simulink model "ParkAssist_Scenario001_cs"  (R2014b)
settings: Solver=ode5  SolverMode=SingleTasking  StartTime=0.0  StopTime=100  FixedStep=1/100  RelTol=1e-3
PreLoadFcn:
  | mbxruntime.callbacks.PreLoadFcn(bdroot);
  | check_NUTS_defined;
  | 
  | assignin('base',['model_closed_' bdroot],false);
  | addpath('../includes_AP');
PostLoadFcn:
  | mbxruntime.callbacks.PostLoadFcn(bdroot);
  | 
  | AP_PlotSpeed;
  | Sim_Stop();
InitFcn:
  | mbxruntime.callbacks.InitFcn(bdroot);
StartFcn:
  | mbxruntime.callbacks.StartFcn(bdroot);
StopFcn:
  | Sim_Stop();
  | 
  | mbxruntime.callbacks.StopFcn(bdroot);
model workspace: external: MAT-File .\ParkAssist_Scenario001_cs_hws.mat (data not in the file)
undefined symbols (not defined in the file or in its folder): mbxruntime, tabledata, warningInitialVelocity, x0
undefined symbols (not defined in the file): ParkAssist_Scenario001_cs_064fd3c184f1b23a, ParkAssist_Scenario001_cs_07cf59fafd9fba2a, ParkAssist_Scenario001_cs_0a672491f171a534, ParkAssist_Scenario001_cs_0b4ad32984af75f4, ParkAssist_Scenario001_cs_0d3d977035912083, ParkAssist_Scenario001_cs_10cfce74ee7f6e2a, ParkAssist_Scenario001_cs_10fa00b62d70eb48, ParkAssist_Scenario001_cs_1412412868c06c72, ParkAssist_Scenario001_cs_1415f498d2c97e5b, ParkAssist_Scenario001_cs_14cdb1b1e9831a61, ParkAssist_Scenario001_cs_17aa22f6296b2219, ParkAssist_Scenario001_cs_182e9fc64682f276, ParkAssist_Scenario001_cs_18d73450bb29fb11, ParkAssist_Scenario001_cs_1d2cd226ded8d576, ParkAssist_Scenario001_cs_1f257bc72917fbbc, ParkAssist_Scenario001_cs_1f636db8464e6ee8, ParkAssist_Scenario001_cs_20111ee9b4fc0884, ParkAssist_Scenario001_cs_20dc177d733a24ce, ParkAssist_Scenario001_cs_216ba491a5d003d6, ParkAssist_Scenario001_cs_23109d51cb4d704e, ParkAssist_Scenario001_cs_269c9790c06f4ab8, ParkAssist_Scenario001_cs_26fe2e7e8db3d6a5, ParkAssist_Scenario001_cs_29ddfbdf1c0505e3, ParkAssist_Scenario001_cs_2a5436d5f4ead3bb, ParkAssist_Scenario001_cs_2bb3c9b455f29773, ParkAssist_Scenario001_cs_2e8c42de3c2a47e4, ParkAssist_Scenario001_cs_31bf8e412bef9025, ParkAssist_Scenario001_cs_346fcd7bf176a778, ParkAssist_Scenario001_cs_3672d2bf8313cd6a, ParkAssist_Scenario001_cs_3741824a7a646254, ParkAssist_Scenario001_cs_39b3d14ce0df0209, ParkAssist_Scenario001_cs_3a61ee37372b31a8, ParkAssist_Scenario001_cs_3c92fe98e00232e8, ParkAssist_Scenario001_cs_3cb2af30b2d7797f, ParkAssist_Scenario001_cs_3cf6ddcf435d426b, ParkAssist_Scenario001_cs_3e68616cf9f62179, ParkAssist_Scenario001_cs_40255007183c2d89, ParkAssist_Scenario001_cs_453862d7bd596598, ParkAssist_Scenario001_cs_456f9ff24294bad4, ParkAssist_Scenario001_cs_45cf167d6b79cbb0, ParkAssist_Scenario001_cs_461748130c9c9c60, ParkAssist_Scenario001_cs_46b365d527226409, ParkAssist_Scenario001_cs_4cef5fe3be802cd9, ParkAssist_Scenario001_cs_4db296735c90de52, ParkAssist_Scenario001_cs_534e2bc3ff1a973e, ParkAssist_Scenario001_cs_55eebfeaa672d93d, ParkAssist_Scenario001_cs_585d6997c12221bd, ParkAssist_Scenario001_cs_5870adf5737dbe97, ParkAssist_Scenario001_cs_59a06d303da3d6df, ParkAssist_Scenario001_cs_59facc8727fc2440, ParkAssist_Scenario001_cs_5a3707b9202e3d67, ParkAssist_Scenario001_cs_5a9d74932f04a2aa, ParkAssist_Scenario001_cs_5b15da5d0cd6c04f, ParkAssist_Scenario001_cs_5cc17ff8d1eedb9f, ParkAssist_Scenario001_cs_5e786d0919c35899, ParkAssist_Scenario001_cs_60157af7bdca7094, ParkAssist_Scenario001_cs_6036a1ff9e25f439, ParkAssist_Scenario001_cs_6071b03654d6c39c, ParkAssist_Scenario001_cs_610f0d4aebe0cae1, ParkAssist_Scenario001_cs_622920b41ce6c5d3 ... (+103)
libraries: PreScanUsefulBlocks x57, PreScanSimulinkLibrary x56, simulink x55, simulink_extras x6
(part 9 of 15)

== system ParkAssist_Scenario001_cs/Audi_A8_1/AP_DEMO/Trigger_&_Display_Subsystem ==
  V [m/s] : Inport
  Gear : Inport  Port=2
  Throttle : Inport  Port=3
  Braking Pressure : Inport  Port=4
  Steering Angle : Inport  Port=5
  DISPLAY : M-S-Function  FunctionName=msfcn_AP_PlotSpeed  Parameters=DisplayFreq PathName
      mask Display:
      | port_label('input',1,'Velocity [km/h]');
      | port_label('input',2,'Gear');
      | port_label('input',3,'Brake Pressure [bar]');
      | port_label('input',4,'Throttle [%]');
      | port_label('input',5,'Steering Angle');
      | port_label('input',6,'Vehicle State');
  Error Check : Subsystem
  Rate Limiter : RateLimiter  RisingSlewLimit=500  FallingSlewLimit=-500  SampleTimeMode=inherited
  Trigger_system : Subsystem
  m/s 2 km/h : Gain  Gain=3.6
  Triggers : Outport
  Trigger2 : Outport  Port=2
  wires:
  Throttle/1 -> DISPLAY/4
  Braking Pressure/1 -> DISPLAY/3
  Steering Angle/1 -> Rate Limiter/1
  Gear/1 -> DISPLAY/2
  m/s 2 km/h/1 -> DISPLAY/1
  Trigger_system/2(Trigger2) -> Trigger2/1
  Trigger_system/1(Triggers) -> Triggers/1, DISPLAY/6
  V [m/s]/1 -> Trigger_system/1(V [m/s]), m/s 2 km/h/1
  Rate Limiter/1 -> DISPLAY/5

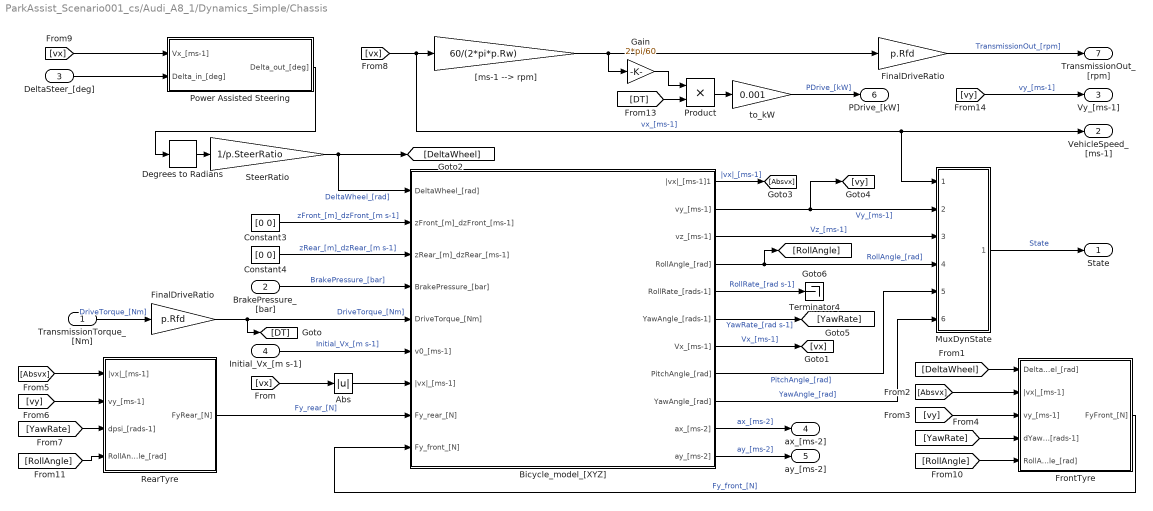
== system ParkAssist_Scenario001_cs/Audi_A8_1/Dynamics_Simple/Chassis ==
  TransmissionTorque_[Nm] : Inport
  BrakePressure_[bar] : Inport  Port=2
  DeltaSteer_[deg] : Inport  Port=3
  Initial_Vx_[m s-1] : Inport  Port=4
  Abs : Abs
  Bicycle_model_[XYZ] : Subsystem
      mask Display: image(imread('Bicycle_model.png'));
  Constant3 : Constant  Value=[0 0]
  Constant4 : Constant  Value=[0 0]
  Degrees to Radians : simulink_extras/Transformations/Degrees to Radians
  FinalDriveRatio : Gain  Gain=p.Rfd  SaturateOnIntegerOverflow=on  OutDataTypeStr=Inherit: Same as input  ParamDataTypeStr=Inherit: Same as input
  "FinalDriveRatio " : Gain  Gain=p.Rfd  SaturateOnIntegerOverflow=on  OutDataTypeStr=Inherit: Same as input  ParamDataTypeStr=Inherit: Same as input
  FrontTyre : Subsystem
      mask Display: image(imread('Tyre.png'));
  Gain : Gain  Gain=2*pi/60
  MuxDynState : Subsystem
  Power Assisted Steering : Subsystem
  Product : Product  RndMeth=Zero
  RearTyre : Subsystem
      mask Display: image(imread('Tyre.png'));
  SteerRatio : Gain  Gain=1/p.SteerRatio
  Terminator4 : Terminator
  "[ms-1 --> rpm]" : Gain  Gain=60/(2*pi*p.Rw)  SaturateOnIntegerOverflow=on  OutDataTypeStr=Inherit: Same as input  ParamDataTypeStr=Inherit: Same as input
  to_kW : Gain  Gain=0.001
  State : Outport
  VehicleSpeed_[ms-1] : Outport  Port=2
  Vy_[ms-1] : Outport  Port=3
  ax_[ms-2] : Outport  Port=4
  ay_[ms-2] : Outport  Port=5
  PDrive_[kW] : Outport  Port=6
  TransmissionOut_[rpm] : Outport  Port=7
  wires:
  [vy] -> Vy_[ms-1]/1  "vy_[ms-1]"
  to_kW/1 -> PDrive_[kW]/1  "PDrive_[kW]"
  Gain/1 -> Product/1
  Bicycle_model_[XYZ]/10(ax_[ms-2]) -> ax_[ms-2]/1  "ax_[ms-2]"
  Product/1 -> to_kW/1
  [DT] -> Product/2
  Bicycle_model_[XYZ]/11(ay_[ms-2]) -> ay_[ms-2]/1  "ay_[ms-2]"
  Abs/1 -> Bicycle_model_[XYZ]/7(|vx|_[ms-1])
  Degrees to Radians/1 -> SteerRatio/1
  [vx] -> Abs/1
  SteerRatio/1 -> [DeltaWheel], Bicycle_model_[XYZ]/1(DeltaWheel_[rad])  "DeltaWheel_[rad]"
  TransmissionTorque_[Nm]/1 -> "FinalDriveRatio "/1  "DriveTorque_[Nm]"
  RearTyre/1(FyRear_[N]) -> Bicycle_model_[XYZ]/8(Fy_rear_[N])  "Fy_rear_[N]"
  FrontTyre/1(FyFront_[N]) -> Bicycle_model_[XYZ]/9(Fy_front_[N])  "Fy_front_[N]"
  Bicycle_model_[XYZ]/1(|vx|_[ms-1]1) -> [Absvx]  "|vx|_[ms-1]"
  Bicycle_model_[XYZ]/2(vy_[ms-1]) -> [vy], MuxDynState/2(vy [ms-1])  "Vy_[ms-1]"
  Bicycle_model_[XYZ]/4(RollAngle_[rad]) -> MuxDynState/4(R [rad]), [RollAngle]  "RollAngle_[rad]"
  Bicycle_model_[XYZ]/6(YawAngle_[rads-1]) -> [YawRate]  "YawRate_[rad s-1]"
  Bicycle_model_[XYZ]/7(Vx_[ms-1]) -> [vx]  "Vx_[ms-1]"
  [DeltaWheel] -> FrontTyre/1(DeltaWheel_[rad])
  [Absvx] -> FrontTyre/2(|vx|_[ms-1])
  [vy] -> FrontTyre/3(vy_[ms-1])
  [YawRate] -> FrontTyre/4(dYawAngle_[rads-1])
  [Absvx] -> RearTyre/1(|vx|_[ms-1])
  [vy] -> RearTyre/2(vy_[ms-1])
  [YawRate] -> RearTyre/3(dpsi_[rads-1])
  Bicycle_model_[XYZ]/3(vz_[ms-1]) -> MuxDynState/3(vz [ms-1])  "Vz_[ms-1]"
  Bicycle_model_[XYZ]/8(PitchAngle_[rad]) -> MuxDynState/5(P [rad])  "PitchAngle_[rad]"
  Bicycle_model_[XYZ]/9(YawAngle_[rad]) -> MuxDynState/6(Y [rad])  "YawAngle_[rad]"
  "[ms-1 --> rpm]"/1 -> Gain/1, FinalDriveRatio/1
  FinalDriveRatio/1 -> TransmissionOut_[rpm]/1  "TransmissionOut_[rpm]"
  [vx] -> "[ms-1 --> rpm]"/1, VehicleSpeed_[ms-1]/1, MuxDynState/1(vx [ms-1])  "vx_[ms-1]"
  [vx] -> Power Assisted Steering/1(Vx_[ms-1])
  DeltaSteer_[deg]/1 -> Power Assisted Steering/2(Delta_in_[deg])
  Power Assisted Steering/1(Delta_out_[deg]) -> Degrees to Radians/1
  [RollAngle] -> FrontTyre/5(RollAngle_[rad])
  [RollAngle] -> RearTyre/4(RollAngle_[rad])
  Constant3/1 -> Bicycle_model_[XYZ]/2(zFront_[m]_dzFront_[ms-1])  "zFront_[m]_dzFront_[m s-1]"
  Constant4/1 -> Bicycle_model_[XYZ]/3(zRear_[m]_dzRear_[ms-1])  "zRear_[m]_dzRear_[m s-1]"
  BrakePressure_[bar]/1 -> Bicycle_model_[XYZ]/4(BrakePressure_[bar])  "BrakePressure_[bar]"
  "FinalDriveRatio "/1 -> Bicycle_model_[XYZ]/5(DriveTorque_[Nm]), [DT]  "DriveTorque_[Nm]"
  Initial_Vx_[m s-1]/1 -> Bicycle_model_[XYZ]/6(v0_[ms-1])  "Initial_Vx_[m s-1]"
  Bicycle_model_[XYZ]/5(RollRate_[rads-1]) -> Terminator4/1  "RollRate_[rad s-1]"
  MuxDynState/1(State) -> State/1  "State"

== system ParkAssist_Scenario001_cs/Audi_A8_1/Dynamics_Simple/Engine ==
  ImpellerTorque_[Nm] : Inport
  Throttle_[%] : Inport  Port=2
  Configurable Subsystem : Subsystem  BlockChoice=Discrete Rate Limiter  mask{ComputationMode=ComputationMode}
      mask prompts: ComputationMode "Compuation mode:"
      mask init:
      | SetComputationMode(gcb,ComputationMode);
      settings: AttributesFormatString=%<BlockChoice>  OpenFcn=BringToFront(gcb);  MemberBlocks=Discrete Rate Limiter,Rate Limiter
      settings: TemplateBlock=|
      | PreScanSimulinkLibrary/Configurable Subsystems/TransferFunction
      | Engine/Configurable
      | Subsystem
  Configurable Subsystem1 : Subsystem  BlockChoice=Discrete-Time Integrator  mask{ComputationMode=ComputationMode}
      mask prompts: ComputationMode "Computation mode:"
      mask init:
      | SetComputationMode(gcb,ComputationMode);
      settings: AttributesFormatString=%<BlockChoice>  OpenFcn=BringToFront(gcb);  MemberBlocks=Discrete-Time Integrator,Integrator
      settings: TemplateBlock=|
      | PreScanSimulinkLibrary/Configurable Subsystems/integral with initial condition and limts
      | for engine/Configurable
      | Subsystem
  EngineTorque : Lookup2D  RowIndex=p.thvec  ColumnIndex=p.nevec  Table=p.emap  InputSameDT=on
  Gain : Gain  Gain=2*pi/60
  Product : Product  RndMeth=Zero
  Sum : Sum  Inputs=-+  SaturateOnIntegerOverflow=on  InputSameDT=on  OutDataTypeStr=Inherit: Same as first input
  engine + impeller inertia : Gain  Gain=1/p.Iei  SaturateOnIntegerOverflow=on  OutDataTypeStr=Inherit: Same as input  ParamDataTypeStr=Inherit: Same as input
  rad|sec2rpm : Gain  Gain=60/2/pi  SaturateOnIntegerOverflow=on  OutDataTypeStr=Inherit: Same as input  ParamDataTypeStr=Inherit: Same as input
  to_kW : Gain  Gain=0.001
  nEngine_[rpm] : Outport  InitialOutput=0
  PEngine_[kW] : Outport  Port=2  InitialOutput=0
  wires:
  rad|sec2rpm/1 -> nEngine_[rpm]/1, EngineTorque/2, Gain/1  "rpm"
  engine + impeller inertia/1 -> Configurable Subsystem1/1(In1)  "rads-2"
  EngineTorque/1 -> Sum/2, Product/2
  Sum/1 -> engine + impeller inertia/1
  Configurable Subsystem1/1(Out1) -> rad|sec2rpm/1  "rads-1"
  Throttle_[%]/1 -> Configurable Subsystem/1(In1)
  ImpellerTorque_[Nm]/1 -> Sum/1
  Configurable Subsystem/1(Out1) -> EngineTorque/1
  Product/1 -> to_kW/1
  Gain/1 -> Product/1
  to_kW/1 -> PEngine_[kW]/1

== system ParkAssist_Scenario001_cs/Audi_A8_1/Dynamics_Simple/Gear: Auto Manual ==
  note: 0; Auto = on // Manual =off
      | 1; Auto = off // Manual =on
  Auto_Manual : Inport
  Manual_Gear : Inport  Port=2
  Auto_Gear : Inport  Port=3
  If : If  IfExpression=u1 == 0
  If Action Subsystem : Subsystem  TreatAsAtomicUnit=on
  If Action Subsystem1 : Subsystem  TreatAsAtomicUnit=on
  Merge : Merge
  Gear : Outport
  wires:
  If Action Subsystem/1(Out1) -> Merge/1
  Auto_Gear/1 -> If Action Subsystem/1(In1)
  If/1 -> If Action Subsystem/Action
  Merge/1 -> Gear/1
  If Action Subsystem1/1(Out1) -> Merge/2
  Manual_Gear/1 -> If Action Subsystem1/1(In1)
  If/2 -> If Action Subsystem1/Action
  Auto_Manual/1 -> If/1

== system ParkAssist_Scenario001_cs/Audi_A8_1/Dynamics_Simple/ShiftLogic ==
  Throttle_[%] : Inport
  GearNr_[-] : Inport  Port=2
  Auto_GearShift : Inport  Port=3
  VehSpeed_[ms-1] : Inport  Port=4
  Add2 : Sum
  Data Type Conversion1 : DataTypeConversion  OutDataTypeStr=double
  Detect Increase1 : simulink/Logic and Bit Operations/Detect Increase  vinit=0.0  InputProcessing=Inherited  OutDataTypeStr=uint8
  Detect Increase : Subsystem
  Gear limitation : Saturate  UpperLimit=p.maxGear  LowerLimit=1
  Gear limitation while shifting : Saturate  UpperLimit=p.maxGear  LowerLimit=1
  GearNeutral : Constant  Value=0
  GearReverse : Constant  Value=-1
  "IC, gear = 1" : Memory  X0=1  InheritSampleTime=on
  If Action Neutral : Subsystem  TreatAsAtomicUnit=on
  If Action Normal : Subsystem  TreatAsAtomicUnit=on
  If Action Reverse : Subsystem  TreatAsAtomicUnit=on
  Memory : Memory  InheritSampleTime=on
  Merge : Merge  Inputs=3
  Relational Operator : RelationalOperator  OutDataTypeStr=boolean
  Relational Operator1 : RelationalOperator  Operator=<=  OutDataTypeStr=boolean
  Shift_Down time : Delay  DelayLength=p.ShiftDown_fac  InputProcessing=Inherited
  Shift_Up time : Delay  DelayLength=p.ShiftUp_fac  InputProcessing=Inherited
  Sum : Sum  Inputs=+-
  interp_down : Lookup2D  RowIndex=p.downth  ColumnIndex=[1:p.maxGear]  Table=p.downtab  LookUpMeth=Interpolation-Use End Values  InputSameDT=on
  interp_up : Lookup2D  RowIndex=p.upth  ColumnIndex=[1:p.maxGear]  Table=p.uptab  LookUpMeth=Interpolation-Use End Values  InputSameDT=on
  reverse/neutral/normal gear : If  IfExpression=u1 == 0  ElseIfExpressions=u1 < 0
  to_ms-1 : Gain  Gain=1/3.6
  "to_ms-1 " : Gain  Gain=1/3.6
  GearNr : Outport
  wires:
  Auto_GearShift/1 -> reverse/neutral/normal gear/1
  "IC, gear = 1"/1 -> If Action Normal/1(In1)
  Merge/1 -> GearNr/1
  If Action Reverse/1(Out1) -> Merge/2
  If Action Neutral/1(Out1) -> Merge/1
  If Action Normal/1(Out1) -> Merge/3
  reverse/neutral/normal gear/3 -> If Action Normal/Action
  reverse/neutral/normal gear/1 -> If Action Neutral/Action
  reverse/neutral/normal gear/2 -> If Action Reverse/Action
  GearReverse/1 -> If Action Reverse/1(In1)
  GearNeutral/1 -> If Action Neutral/1(In1)
  Shift_Down time/1 -> Sum/2
  Shift_Up time/1 -> Sum/1
  Detect Increase/1(Out1) -> Shift_Up time/1
  Data Type Conversion1/1 -> Shift_Down time/1
  Detect Increase1/1 -> Data Type Conversion1/1
  Sum/1 -> Add2/1
  Memory/1 -> Add2/2  "GearNr_[-]"
  Add2/1 -> Gear limitation while shifting/1
  Gear limitation while shifting/1 -> "IC, gear = 1"/1, Memory/1  "GearNr_[-]"
  Throttle_[%]/1 -> interp_down/1, interp_up/1
  Relational Operator/1 -> Detect Increase/2(In2)
  Relational Operator1/1 -> Detect Increase1/1
  interp_down/1 -> "to_ms-1 "/1
  VehSpeed_[ms-1]/1 -> Relational Operator/1, Relational Operator1/1
  interp_up/1 -> to_ms-1/1
  Gear limitation/1 -> interp_down/2, interp_up/2, Detect Increase/1(GearNr_[-])
  GearNr_[-]/1 -> Gear limitation/1
  to_ms-1/1 -> Relational Operator/2
  "to_ms-1 "/1 -> Relational Operator1/2

== system ParkAssist_Scenario001_cs/Audi_A8_1/Dynamics_Simple/Transmission ==
  nEngine_[rpm] : Inport
  GearNr_[-] : Inport  Port=2
  n_TransmissionOut_[rpm] : Inport  Port=3
  Torque_Converter : Subsystem
      mask Display: image(imread('TorqueConverter.png'));
  Transmission_Ratio : Subsystem
  Viscous coupling : Lookup  InputValues=[-5:0.1:5]*p.m/4  Table=p.m/4*tanh([-5:0.1:5])
  ImpellerTorque_[Nm] : Outport  InitialOutput=0
  TransmissionTorque_[Nm] : Outport  Port=2  InitialOutput=0
  wires:
  Torque_Converter/2(TurbineTorque_[Nm]) -> Viscous coupling/1  "Converter_Torque_[Nm]"
  Transmission_Ratio/2(nTransmissionIn_[rpm]) -> Torque_Converter/2(nTransmission_[rpm])
  nEngine_[rpm]/1 -> Torque_Converter/1(nEngine_[rpm])
  GearNr_[-]/1 -> Transmission_Ratio/2(GearNr_[-]), Torque_Converter/3(Gear nr)
  n_TransmissionOut_[rpm]/1 -> Transmission_Ratio/3(nTransmissionOut_[rpm])
  Torque_Converter/1(ImpellerTorque_[Nm]) -> ImpellerTorque_[Nm]/1
  Transmission_Ratio/1(tTransmissionOut_[Nm]) -> TransmissionTorque_[Nm]/1
  Viscous coupling/1 -> Transmission_Ratio/1(tTransmissionIn_[Nm])

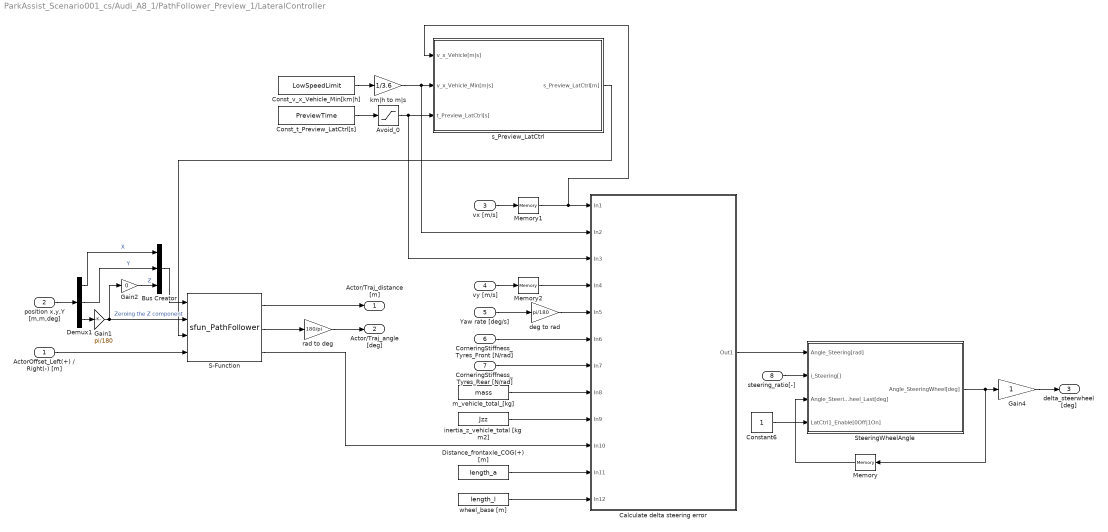
== system ParkAssist_Scenario001_cs/Audi_A8_1/PathFollower_Preview_1/LateralController ==
  ActorOffset_Left(+) / Right(-) [m] : Inport
  position x,y,Y [m,m,deg] : Inport  Port=2
  vx [m/s] : Inport  Port=3
  vy [m/s] : Inport  Port=4
  Yaw rate [deg/s] : Inport  Port=5
  CorneringStiffness_Tyres_Front [N/rad] : Inport  Port=6
  CorneringStiffness_Tyres_Rear [N/rad] : Inport  Port=7
  steering_ratio[-] : Inport  Port=8
  Avoid_0 : Saturate  UpperLimit=1000  LowerLimit=0.1
  Bus Creator : BusCreator  Inputs='X','Y','Z'  OutDataTypeStr=Bus: PRESCAN_XYZ_DATA
  Calculate delta steering error : Subsystem
      mask Display:
      | port_label('input', 1, 'v_x_vehicle [m/s]')
      | port_label('input', 2, 'v_x_vehicle_Min [m/s]')
      | port_label('input', 3, 't_Preview_LatCtrl [s]')
      | port_label('input', 4, 'v_y_vehicle [m/s]')
      | port_label('input', 5, 'yawrate_vehicle [rad/sec]')
      | port_label('input', 6, 'CorneringStiffness_Tyres_Front [N/rad]')
      | port_label('input', 7, 'CorneringStiffness_Tyres_Rear [N/rad]')
      | port_label('input', 8, 'm_vehicle_total [kg]')
      | port_label('input', 9, 'inertia_z_vehicle_total [kg m2]')
      | port_label('input', 10, 'e_Lat [m]')
      | port_label('input', 11, 'Distance_frontaxle_COG(+) [m]')
      | port_label('input', 12, 'wheel_base [m]')
      | port_label('output', 1, 'delta_steeringwheel [rad]')
  Const_t_Preview_LatCtrl[s] : Constant  Value=PreviewTime  SampleTime=CSSampleTime
  Const_v_x_Vehicle_Min[km|h] : Constant  Value=LowSpeedLimit  SampleTime=CSSampleTime
  Constant6 : Constant  SampleTime=CSSampleTime
  Demux1 : Demux  Outputs=3
  Distance_frontaxle_COG(+) [m] : Constant  Value=length_a  SampleTime=CSSampleTime
  Gain1 : Gain  Gain=pi/180
  Gain2 : Gain  Gain=0
  Gain4 : Gain
  Memory : Memory  InheritSampleTime=on
  Memory1 : Memory  InheritSampleTime=on
  Memory2 : Memory  InheritSampleTime=on
  S-Function : S-Function  FunctionName=sfun_PathFollower  Parameters=PathUniqueID,-1  EnableBusSupport=off
  SteeringWheelAngle : Subsystem
  deg to rad : Gain  Gain=pi/180
  inertia_z_vehicle_total [kg m2] : Constant  Value=Jzz  SampleTime=CSSampleTime
  km|h to m|s : Gain  Gain=1/3.6
  m_vehicle_total_[kg] : Constant  Value=mass  SampleTime=CSSampleTime
  rad to deg : Gain  Gain=180/pi
  s_Preview_LatCtrl : Subsystem
  wheel_base [m] : Constant  Value=length_l  SampleTime=CSSampleTime
  Actor/Traj_distance [m] : Outport
  Actor/Traj_angle [deg] : Outport  Port=2
  delta_steerwheel [deg] : Outport  Port=3
  wires:
  Gain2/1 -> Bus Creator/3  "Z"
  Bus Creator/1 -> S-Function/1
  Demux1/2 -> Bus Creator/2  "Y"
  Demux1/1 -> Bus Creator/1  "X"
  s_Preview_LatCtrl/1(s_Preview_LatCtrl[m]) -> S-Function/3
  rad to deg/1 -> Actor/Traj_angle [deg]/1
  km|h to m|s/1 -> Calculate delta steering error/2(In2), s_Preview_LatCtrl/2(v_x_Vehicle_Min[m|s])
  ActorOffset_Left(+) / Right(-) [m]/1 -> S-Function/4
  S-Function/2 -> rad to deg/1
  S-Function/1 -> Actor/Traj_distance [m]/1
  Calculate delta steering error/1(Out1) -> SteeringWheelAngle/1(Angle_Steering[rad])
  vx [m/s]/1 -> Memory1/1
  vy [m/s]/1 -> Memory2/1
  CorneringStiffness_Tyres_Front [N/rad]/1 -> Calculate delta steering error/6(In6)
  m_vehicle_total_[kg]/1 -> Calculate delta steering error/8(In8)
  inertia_z_vehicle_total [kg m2]/1 -> Calculate delta steering error/9(In9)
  steering_ratio[-]/1 -> SteeringWheelAngle/2(i_Steering[])
  SteeringWheelAngle/1(Angle_SteeringWheel[deg]) -> Gain4/1, Memory/1
  Memory/1 -> SteeringWheelAngle/3(Angle_SteeringWheel_Last[deg])
  Constant6/1 -> SteeringWheelAngle/4(LatCtrl1_Enable[0Off|1On])
  Avoid_0/1 -> Calculate delta steering error/3(In3), s_Preview_LatCtrl/3(t_Preview_LatCtrl[s])
  Const_v_x_Vehicle_Min[km|h]/1 -> km|h to m|s/1
  Const_t_Preview_LatCtrl[s]/1 -> Avoid_0/1
  Gain4/1 -> delta_steerwheel [deg]/1
  Distance_frontaxle_COG(+) [m]/1 -> Calculate delta steering error/11(In11)
  CorneringStiffness_Tyres_Rear [N/rad]/1 -> Calculate delta steering error/7(In7)
  Yaw rate [deg/s]/1 -> deg to rad/1
  deg to rad/1 -> Calculate delta steering error/5(In5)
  Gain1/1 -> Gain2/1, S-Function/2  "Zeroing the Z component"
  Demux1/3 -> Gain1/1
  position x,y,Y [m,m,deg]/1 -> Demux1/1
  wheel_base [m]/1 -> Calculate delta steering error/12(In12)
  S-Function/3 -> Calculate delta steering error/10(In10)
  Memory1/1 -> Calculate delta steering error/1(In1), s_Preview_LatCtrl/1(v_x_Vehicle[m|s])
  Memory2/1 -> Calculate delta steering error/4(In4)

== system ParkAssist_Scenario001_cs/Audi_A8_1/PathFollower_Preview_1/LongitudinalController ==
  v_actual [m/s] : Inport
  Desired Velocity [m/s] : Inport  Port=2
  Initial Velocity [m/s] : Inport  Port=3
  Check_Initial_Velocity : Subsystem
  Demux : Demux  Outputs=3
  GearNormal : Constant
  "GearNormal " : Constant
  If Desired Velocity = 0 : Subsystem  TreatAsAtomicUnit=on
  If Desired Velocity ~= 0 : Subsystem  TreatAsAtomicUnit=on
  Memory External IC : Subsystem
  Merge : Merge
  Mux : Mux  Inputs=3
  Mux2 : Mux  Inputs=3
  Sum4 : Sum  Inputs=|+-
  if : If  IfExpression=u1 == 0  SampleTime=CSSampleTime
  throttle [%] : Outport
  brake pressure [bar] : Outport  Port=2
  v0 [m/s] : Outport  Port=3
  Auto_GearShift : Outport  Port=4
  wires:
  v_actual [m/s]/1 -> Check_Initial_Velocity/1(" v_actual_[m|s]"), Memory External IC/1(u)
  Memory External IC/1(y) -> Sum4/2
  Sum4/1 -> If Desired Velocity ~= 0/2(Desired Velocity [m/s])
  Desired Velocity [m/s]/1 -> if/1, Sum4/1
  Initial Velocity [m/s]/1 -> Check_Initial_Velocity/2(Initial_Velocity_[m|s]), Memory External IC/2(IC), v0 [m/s]/1
  GearNormal/1 -> If Desired Velocity = 0/1(In1)
  Merge/1 -> Demux/1
  If Desired Velocity = 0/1(throttle [%]) -> Mux/1
  If Desired Velocity = 0/2(brake pressure [bar]) -> Mux/2
  Mux2/1 -> Merge/2
  Mux/1 -> Merge/1
  Demux/1 -> throttle [%]/1
  Demux/2 -> brake pressure [bar]/1
  Demux/3 -> Auto_GearShift/1
  "GearNormal "/1 -> If Desired Velocity ~= 0/1(In1)
  If Desired Velocity = 0/3(Auto_GearShift) -> Mux/3
  if/2 -> If Desired Velocity ~= 0/Action
  if/1 -> If Desired Velocity = 0/Action
  If Desired Velocity ~= 0/1(throttle [%]) -> Mux2/1
  If Desired Velocity ~= 0/2(brake pressure [bar]) -> Mux2/2
  If Desired Velocity ~= 0/3(Auto_GearShift) -> Mux2/3

== system ParkAssist_Scenario001_cs/Audi_A8_1/SELF_Demux/compas converter ==
  rotz [rad] : Inport
  cart2compas : Subsystem
  rad2deg : Gain  Gain=180/pi
  heading [deg] : Outport
  wires:
  rad2deg/1 -> cart2compas/1(Angle [deg])
  rotz [rad]/1 -> rad2deg/1
  cart2compas/1(heading [deg]) -> heading [deg]/1

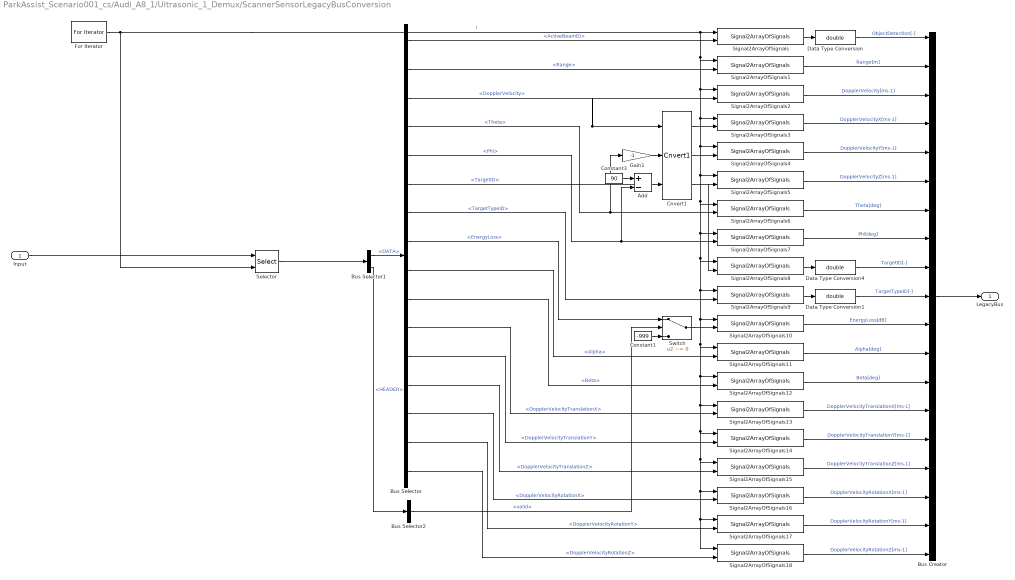
== system ParkAssist_Scenario001_cs/Audi_A8_1/Ultrasonic_1_Demux/ScannerSensorLegacyBusConversion ==
  Input : Inport
  Add : Sum  Inputs=+-
  Bus Creator : BusCreator  Inputs=19
  Bus Selector : BusSelector  OutputSignals=ActiveBeamID,Range,DopplerVelocity,Theta,Phi,TargetID,TargetTypeID,EnergyLoss,Alpha,Beta,DopplerVelocityTranslationX,DopplerVelocityTranslationY,DopplerVelocityTranslationZ,DopplerVelocityRotationX,DopplerVelocityRotationY,DopplerVelocityRotationZ
  Bus Selector1 : BusSelector  OutputSignals=DATA,HEADER
  Bus Selector2 : BusSelector  OutputSignals=valid
  Cnvert1 : PreScanSimulinkLibrary/Cnvert1
  Constant1 : Constant  Value=-999
  Constant3 : Constant  Value=90
  Data Type Conversion : DataTypeConversion  OutDataTypeStr=double  LockScale=on
  Data Type Conversion1 : DataTypeConversion  OutDataTypeStr=double  LockScale=on
  Data Type Conversion4 : DataTypeConversion  OutDataTypeStr=double  LockScale=on
  For Iterator : ForIterator  ResetStates=reset  IterationLimit=MAXMESSAGES
  Gain1 : Gain  Gain=-1
  Selector : Selector  InputPortWidth=MAXMESSAGES  IndexOptions=Index vector (port)  Indices=[1 3]
  Signal2ArrayOfSignals{,1..18} (19 alike) : PreScanUsefulBlocks/Signal2ArrayOfSignals  VECTORLENGTH=MAXMESSAGES
  Switch : Switch  Criteria=u2 ~= 0  Threshold=1
  LegacyBus : Outport
  wires:
  Bus Creator/1 -> LegacyBus/1
  Signal2ArrayOfSignals12/1 -> Bus Creator/13  "Beta[deg]"
  Signal2ArrayOfSignals11/1 -> Bus Creator/12  "Alpha[deg]"
  Signal2ArrayOfSignals10/1 -> Bus Creator/11  "EnergyLoss[dB]"
  Data Type Conversion1/1 -> Bus Creator/10  "TargetTypeID[-]"
  Data Type Conversion4/1 -> Bus Creator/9  "TargetID[-]"
  Signal2ArrayOfSignals7/1 -> Bus Creator/8  "Phi[deg]"
  Signal2ArrayOfSignals6/1 -> Bus Creator/7  "Theta[deg]"
  Signal2ArrayOfSignals5/1 -> Bus Creator/6  "DopplerVelocityZ[ms-1]"
  Signal2ArrayOfSignals4/1 -> Bus Creator/5  "DopplerVelocityY[ms-1]"
  Signal2ArrayOfSignals3/1 -> Bus Creator/4  "DopplerVelocityX[ms-1]"
  Signal2ArrayOfSignals2/1 -> Bus Creator/3  "DopplerVelocity[ms-1]"
  Signal2ArrayOfSignals1/1 -> Bus Creator/2  "Range[m]"
  Data Type Conversion/1 -> Bus Creator/1  "ObjectDetection[-]"
  Signal2ArrayOfSignals9/1 -> Data Type Conversion1/1
  Bus Selector2/1 -> Switch/2  "<valid>"
  Bus Selector1/2 -> Bus Selector2/1  "<HEADER>"
  Bus Selector1/1 -> Bus Selector/1  "<DATA>"
  Switch/1 -> Signal2ArrayOfSignals10/2
  Constant1/1 -> Switch/3
  Bus Selector/8 -> Switch/1  "<EnergyLoss>"
  Selector/1 -> Bus Selector1/1
  Constant3/1 -> Add/1
  Add/1 -> Cnvert1/3
  Gain1/1 -> Cnvert1/2
  Cnvert1/3 -> Signal2ArrayOfSignals5/2
  Cnvert1/2 -> Signal2ArrayOfSignals4/2
  Cnvert1/1 -> Signal2ArrayOfSignals3/2
  Signal2ArrayOfSignals8/1 -> Data Type Conversion4/1
  Bus Selector/1 -> Signal2ArrayOfSignals/2  "<ActiveBeamID>"
  Bus Selector/2 -> Signal2ArrayOfSignals1/2  "<Range>"
  Bus Selector/3 -> Signal2ArrayOfSignals2/2, Cnvert1/1  "<DopplerVelocity>"
  Bus Selector/4 -> Signal2ArrayOfSignals6/2, Gain1/1  "<Theta>"
  Bus Selector/5 -> Signal2ArrayOfSignals7/2, Add/2  "<Phi>"
  Bus Selector/6 -> Signal2ArrayOfSignals8/2  "<TargetID>"
  Bus Selector/7 -> Signal2ArrayOfSignals9/2  "<TargetTypeID>"
  Bus Selector/9 -> Signal2ArrayOfSignals11/2  "<Alpha>"
  Bus Selector/10 -> Signal2ArrayOfSignals12/2  "<Beta>"
  Signal2ArrayOfSignals/1 -> Data Type Conversion/1
  For Iterator/1 -> Signal2ArrayOfSignals11/1, Signal2ArrayOfSignals12/1, Signal2ArrayOfSignals13/1, Signal2ArrayOfSignals14/1, Signal2ArrayOfSignals15/1, Signal2ArrayOfSignals16/1, Signal2ArrayOfSignals17/1, Signal2ArrayOfSignals18/1, Signal2ArrayOfSignals10/1, Signal2ArrayOfSignals9/1, Signal2ArrayOfSignals8/1, Signal2ArrayOfSignals7/1, Signal2ArrayOfSignals6/1, Signal2ArrayOfSignals5/1, Signal2ArrayOfSignals4/1, Signal2ArrayOfSignals3/1, Signal2ArrayOfSignals2/1, Signal2ArrayOfSignals1/1, Signal2ArrayOfSignals/1, Selector/2  "i"
  Input/1 -> Selector/1
  Bus Selector/11 -> Signal2ArrayOfSignals13/2  "<DopplerVelocityTranslationX>"
  Bus Selector/12 -> Signal2ArrayOfSignals14/2  "<DopplerVelocityTranslationY>"
  Bus Selector/13 -> Signal2ArrayOfSignals15/2  "<DopplerVelocityTranslationZ>"
  Bus Selector/14 -> Signal2ArrayOfSignals16/2  "<DopplerVelocityRotationX>"
  Bus Selector/15 -> Signal2ArrayOfSignals17/2  "<DopplerVelocityRotationY>"
  Bus Selector/16 -> Signal2ArrayOfSignals18/2  "<DopplerVelocityRotationZ>"
  Signal2ArrayOfSignals13/1 -> Bus Creator/14  "DopplerVelocityTranslationX[ms-1]"
  Signal2ArrayOfSignals14/1 -> Bus Creator/15  "DopplerVelocityTranslationY[ms-1]"
  Signal2ArrayOfSignals15/1 -> Bus Creator/16  "DopplerVelocityTranslationZ[ms-1]"
  Signal2ArrayOfSignals16/1 -> Bus Creator/17  "DopplerVelocityRotationX[ms-1]"
  Signal2ArrayOfSignals17/1 -> Bus Creator/18  "DopplerVelocityRotationY[ms-1]"
  Signal2ArrayOfSignals18/1 -> Bus Creator/19  "DopplerVelocityRotationZ[ms-1]"

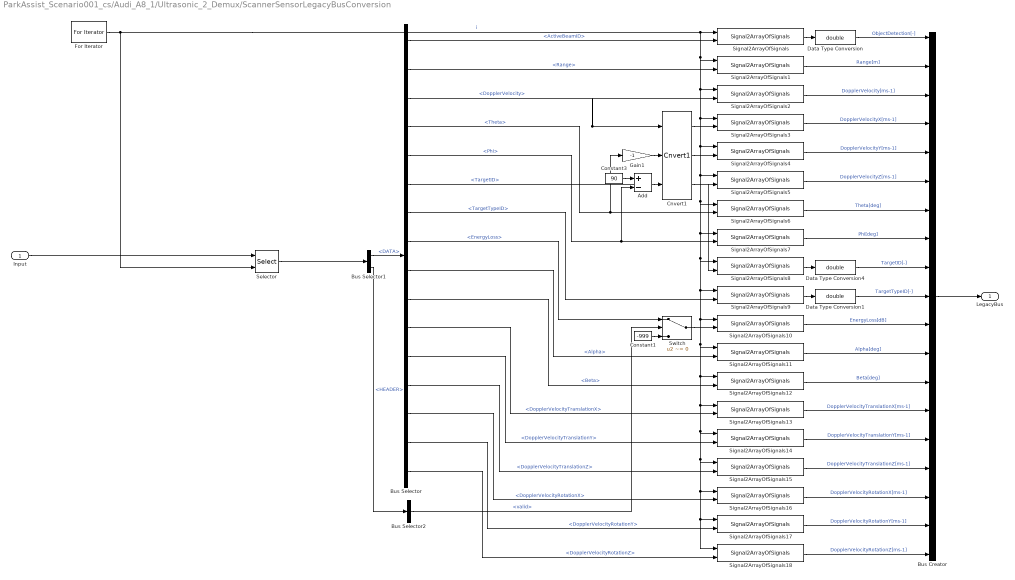
== system ParkAssist_Scenario001_cs/Audi_A8_1/Ultrasonic_2_Demux/ScannerSensorLegacyBusConversion ==
  Input : Inport
  Add : Sum  Inputs=+-
  Bus Creator : BusCreator  Inputs=19
  Bus Selector : BusSelector  OutputSignals=ActiveBeamID,Range,DopplerVelocity,Theta,Phi,TargetID,TargetTypeID,EnergyLoss,Alpha,Beta,DopplerVelocityTranslationX,DopplerVelocityTranslationY,DopplerVelocityTranslationZ,DopplerVelocityRotationX,DopplerVelocityRotationY,DopplerVelocityRotationZ
  Bus Selector1 : BusSelector  OutputSignals=DATA,HEADER
  Bus Selector2 : BusSelector  OutputSignals=valid
  Cnvert1 : PreScanSimulinkLibrary/Cnvert1
  Constant1 : Constant  Value=-999
  Constant3 : Constant  Value=90
  Data Type Conversion : DataTypeConversion  OutDataTypeStr=double  LockScale=on
  Data Type Conversion1 : DataTypeConversion  OutDataTypeStr=double  LockScale=on
  Data Type Conversion4 : DataTypeConversion  OutDataTypeStr=double  LockScale=on
  For Iterator : ForIterator  ResetStates=reset  IterationLimit=MAXMESSAGES
  Gain1 : Gain  Gain=-1
  Selector : Selector  InputPortWidth=MAXMESSAGES  IndexOptions=Index vector (port)  Indices=[1 3]
  Signal2ArrayOfSignals{,1..18} (19 alike) : PreScanUsefulBlocks/Signal2ArrayOfSignals  VECTORLENGTH=MAXMESSAGES
  Switch : Switch  Criteria=u2 ~= 0  Threshold=1
  LegacyBus : Outport
  wires:
  Bus Creator/1 -> LegacyBus/1
  Signal2ArrayOfSignals12/1 -> Bus Creator/13  "Beta[deg]"
  Signal2ArrayOfSignals11/1 -> Bus Creator/12  "Alpha[deg]"
  Signal2ArrayOfSignals10/1 -> Bus Creator/11  "EnergyLoss[dB]"
  Data Type Conversion1/1 -> Bus Creator/10  "TargetTypeID[-]"
  Data Type Conversion4/1 -> Bus Creator/9  "TargetID[-]"
  Signal2ArrayOfSignals7/1 -> Bus Creator/8  "Phi[deg]"
  Signal2ArrayOfSignals6/1 -> Bus Creator/7  "Theta[deg]"
  Signal2ArrayOfSignals5/1 -> Bus Creator/6  "DopplerVelocityZ[ms-1]"
  Signal2ArrayOfSignals4/1 -> Bus Creator/5  "DopplerVelocityY[ms-1]"
  Signal2ArrayOfSignals3/1 -> Bus Creator/4  "DopplerVelocityX[ms-1]"
  Signal2ArrayOfSignals2/1 -> Bus Creator/3  "DopplerVelocity[ms-1]"
  Signal2ArrayOfSignals1/1 -> Bus Creator/2  "Range[m]"
  Data Type Conversion/1 -> Bus Creator/1  "ObjectDetection[-]"
  Signal2ArrayOfSignals9/1 -> Data Type Conversion1/1
  Bus Selector2/1 -> Switch/2  "<valid>"
  Bus Selector1/2 -> Bus Selector2/1  "<HEADER>"
  Bus Selector1/1 -> Bus Selector/1  "<DATA>"
  Switch/1 -> Signal2ArrayOfSignals10/2
  Constant1/1 -> Switch/3
  Bus Selector/8 -> Switch/1  "<EnergyLoss>"
  Selector/1 -> Bus Selector1/1
  Constant3/1 -> Add/1
  Add/1 -> Cnvert1/3
  Gain1/1 -> Cnvert1/2
  Cnvert1/3 -> Signal2ArrayOfSignals5/2
  Cnvert1/2 -> Signal2ArrayOfSignals4/2
  Cnvert1/1 -> Signal2ArrayOfSignals3/2
  Signal2ArrayOfSignals8/1 -> Data Type Conversion4/1
  Bus Selector/1 -> Signal2ArrayOfSignals/2  "<ActiveBeamID>"
  Bus Selector/2 -> Signal2ArrayOfSignals1/2  "<Range>"
  Bus Selector/3 -> Signal2ArrayOfSignals2/2, Cnvert1/1  "<DopplerVelocity>"
  Bus Selector/4 -> Signal2ArrayOfSignals6/2, Gain1/1  "<Theta>"
  Bus Selector/5 -> Signal2ArrayOfSignals7/2, Add/2  "<Phi>"
  Bus Selector/6 -> Signal2ArrayOfSignals8/2  "<TargetID>"
  Bus Selector/7 -> Signal2ArrayOfSignals9/2  "<TargetTypeID>"
  Bus Selector/9 -> Signal2ArrayOfSignals11/2  "<Alpha>"
  Bus Selector/10 -> Signal2ArrayOfSignals12/2  "<Beta>"
  Signal2ArrayOfSignals/1 -> Data Type Conversion/1
  For Iterator/1 -> Signal2ArrayOfSignals11/1, Signal2ArrayOfSignals12/1, Signal2ArrayOfSignals13/1, Signal2ArrayOfSignals14/1, Signal2ArrayOfSignals15/1, Signal2ArrayOfSignals16/1, Signal2ArrayOfSignals17/1, Signal2ArrayOfSignals18/1, Signal2ArrayOfSignals10/1, Signal2ArrayOfSignals9/1, Signal2ArrayOfSignals8/1, Signal2ArrayOfSignals7/1, Signal2ArrayOfSignals6/1, Signal2ArrayOfSignals5/1, Signal2ArrayOfSignals4/1, Signal2ArrayOfSignals3/1, Signal2ArrayOfSignals2/1, Signal2ArrayOfSignals1/1, Signal2ArrayOfSignals/1, Selector/2  "i"
  Input/1 -> Selector/1
  Bus Selector/11 -> Signal2ArrayOfSignals13/2  "<DopplerVelocityTranslationX>"
  Bus Selector/12 -> Signal2ArrayOfSignals14/2  "<DopplerVelocityTranslationY>"
  Bus Selector/13 -> Signal2ArrayOfSignals15/2  "<DopplerVelocityTranslationZ>"
  Bus Selector/14 -> Signal2ArrayOfSignals16/2  "<DopplerVelocityRotationX>"
  Bus Selector/15 -> Signal2ArrayOfSignals17/2  "<DopplerVelocityRotationY>"
  Bus Selector/16 -> Signal2ArrayOfSignals18/2  "<DopplerVelocityRotationZ>"
  Signal2ArrayOfSignals13/1 -> Bus Creator/14  "DopplerVelocityTranslationX[ms-1]"
  Signal2ArrayOfSignals14/1 -> Bus Creator/15  "DopplerVelocityTranslationY[ms-1]"
  Signal2ArrayOfSignals15/1 -> Bus Creator/16  "DopplerVelocityTranslationZ[ms-1]"
  Signal2ArrayOfSignals16/1 -> Bus Creator/17  "DopplerVelocityRotationX[ms-1]"
  Signal2ArrayOfSignals17/1 -> Bus Creator/18  "DopplerVelocityRotationY[ms-1]"
  Signal2ArrayOfSignals18/1 -> Bus Creator/19  "DopplerVelocityRotationZ[ms-1]"

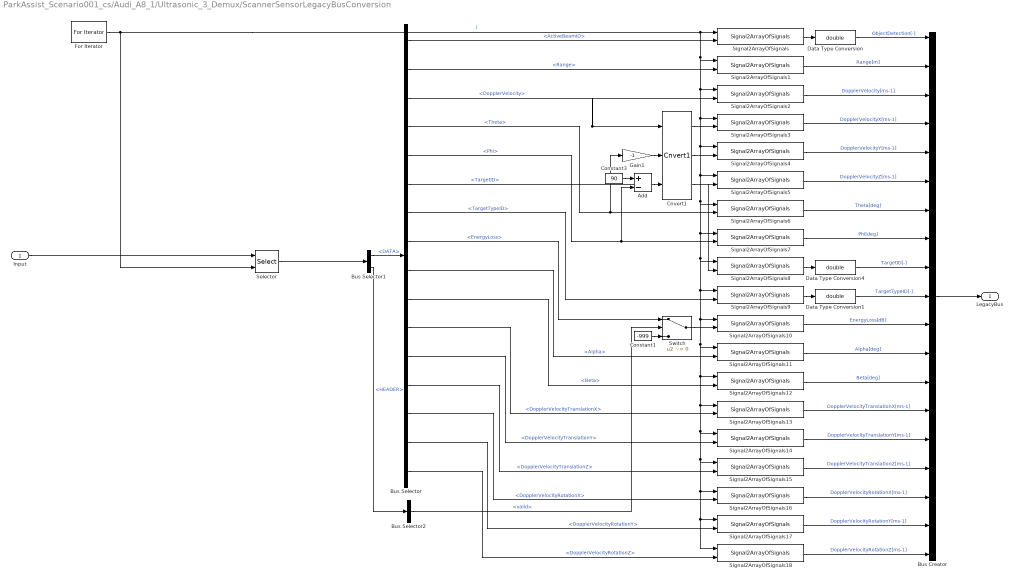
== system ParkAssist_Scenario001_cs/Audi_A8_1/Ultrasonic_3_Demux/ScannerSensorLegacyBusConversion ==
  Input : Inport
  Add : Sum  Inputs=+-
  Bus Creator : BusCreator  Inputs=19
  Bus Selector : BusSelector  OutputSignals=ActiveBeamID,Range,DopplerVelocity,Theta,Phi,TargetID,TargetTypeID,EnergyLoss,Alpha,Beta,DopplerVelocityTranslationX,DopplerVelocityTranslationY,DopplerVelocityTranslationZ,DopplerVelocityRotationX,DopplerVelocityRotationY,DopplerVelocityRotationZ
  Bus Selector1 : BusSelector  OutputSignals=DATA,HEADER
  Bus Selector2 : BusSelector  OutputSignals=valid
  Cnvert1 : PreScanSimulinkLibrary/Cnvert1
  Constant1 : Constant  Value=-999
  Constant3 : Constant  Value=90
  Data Type Conversion : DataTypeConversion  OutDataTypeStr=double  LockScale=on
  Data Type Conversion1 : DataTypeConversion  OutDataTypeStr=double  LockScale=on
  Data Type Conversion4 : DataTypeConversion  OutDataTypeStr=double  LockScale=on
  For Iterator : ForIterator  ResetStates=reset  IterationLimit=MAXMESSAGES
  Gain1 : Gain  Gain=-1
  Selector : Selector  InputPortWidth=MAXMESSAGES  IndexOptions=Index vector (port)  Indices=[1 3]
  Signal2ArrayOfSignals{,1..18} (19 alike) : PreScanUsefulBlocks/Signal2ArrayOfSignals  VECTORLENGTH=MAXMESSAGES
  Switch : Switch  Criteria=u2 ~= 0  Threshold=1
  LegacyBus : Outport
  wires:
  Bus Creator/1 -> LegacyBus/1
  Signal2ArrayOfSignals12/1 -> Bus Creator/13  "Beta[deg]"
  Signal2ArrayOfSignals11/1 -> Bus Creator/12  "Alpha[deg]"
  Signal2ArrayOfSignals10/1 -> Bus Creator/11  "EnergyLoss[dB]"
  Data Type Conversion1/1 -> Bus Creator/10  "TargetTypeID[-]"
  Data Type Conversion4/1 -> Bus Creator/9  "TargetID[-]"
  Signal2ArrayOfSignals7/1 -> Bus Creator/8  "Phi[deg]"
  Signal2ArrayOfSignals6/1 -> Bus Creator/7  "Theta[deg]"
  Signal2ArrayOfSignals5/1 -> Bus Creator/6  "DopplerVelocityZ[ms-1]"
  Signal2ArrayOfSignals4/1 -> Bus Creator/5  "DopplerVelocityY[ms-1]"
  Signal2ArrayOfSignals3/1 -> Bus Creator/4  "DopplerVelocityX[ms-1]"
  Signal2ArrayOfSignals2/1 -> Bus Creator/3  "DopplerVelocity[ms-1]"
  Signal2ArrayOfSignals1/1 -> Bus Creator/2  "Range[m]"
  Data Type Conversion/1 -> Bus Creator/1  "ObjectDetection[-]"
  Signal2ArrayOfSignals9/1 -> Data Type Conversion1/1
  Bus Selector2/1 -> Switch/2  "<valid>"
  Bus Selector1/2 -> Bus Selector2/1  "<HEADER>"
  Bus Selector1/1 -> Bus Selector/1  "<DATA>"
  Switch/1 -> Signal2ArrayOfSignals10/2
  Constant1/1 -> Switch/3
  Bus Selector/8 -> Switch/1  "<EnergyLoss>"
  Selector/1 -> Bus Selector1/1
  Constant3/1 -> Add/1
  Add/1 -> Cnvert1/3
  Gain1/1 -> Cnvert1/2
  Cnvert1/3 -> Signal2ArrayOfSignals5/2
  Cnvert1/2 -> Signal2ArrayOfSignals4/2
  Cnvert1/1 -> Signal2ArrayOfSignals3/2
  Signal2ArrayOfSignals8/1 -> Data Type Conversion4/1
  Bus Selector/1 -> Signal2ArrayOfSignals/2  "<ActiveBeamID>"
  Bus Selector/2 -> Signal2ArrayOfSignals1/2  "<Range>"
  Bus Selector/3 -> Signal2ArrayOfSignals2/2, Cnvert1/1  "<DopplerVelocity>"
  Bus Selector/4 -> Signal2ArrayOfSignals6/2, Gain1/1  "<Theta>"
  Bus Selector/5 -> Signal2ArrayOfSignals7/2, Add/2  "<Phi>"
  Bus Selector/6 -> Signal2ArrayOfSignals8/2  "<TargetID>"
  Bus Selector/7 -> Signal2ArrayOfSignals9/2  "<TargetTypeID>"
  Bus Selector/9 -> Signal2ArrayOfSignals11/2  "<Alpha>"
  Bus Selector/10 -> Signal2ArrayOfSignals12/2  "<Beta>"
  Signal2ArrayOfSignals/1 -> Data Type Conversion/1
  For Iterator/1 -> Signal2ArrayOfSignals11/1, Signal2ArrayOfSignals12/1, Signal2ArrayOfSignals13/1, Signal2ArrayOfSignals14/1, Signal2ArrayOfSignals15/1, Signal2ArrayOfSignals16/1, Signal2ArrayOfSignals17/1, Signal2ArrayOfSignals18/1, Signal2ArrayOfSignals10/1, Signal2ArrayOfSignals9/1, Signal2ArrayOfSignals8/1, Signal2ArrayOfSignals7/1, Signal2ArrayOfSignals6/1, Signal2ArrayOfSignals5/1, Signal2ArrayOfSignals4/1, Signal2ArrayOfSignals3/1, Signal2ArrayOfSignals2/1, Signal2ArrayOfSignals1/1, Signal2ArrayOfSignals/1, Selector/2  "i"
  Input/1 -> Selector/1
  Bus Selector/11 -> Signal2ArrayOfSignals13/2  "<DopplerVelocityTranslationX>"
  Bus Selector/12 -> Signal2ArrayOfSignals14/2  "<DopplerVelocityTranslationY>"
  Bus Selector/13 -> Signal2ArrayOfSignals15/2  "<DopplerVelocityTranslationZ>"
  Bus Selector/14 -> Signal2ArrayOfSignals16/2  "<DopplerVelocityRotationX>"
  Bus Selector/15 -> Signal2ArrayOfSignals17/2  "<DopplerVelocityRotationY>"
  Bus Selector/16 -> Signal2ArrayOfSignals18/2  "<DopplerVelocityRotationZ>"
  Signal2ArrayOfSignals13/1 -> Bus Creator/14  "DopplerVelocityTranslationX[ms-1]"
  Signal2ArrayOfSignals14/1 -> Bus Creator/15  "DopplerVelocityTranslationY[ms-1]"
  Signal2ArrayOfSignals15/1 -> Bus Creator/16  "DopplerVelocityTranslationZ[ms-1]"
  Signal2ArrayOfSignals16/1 -> Bus Creator/17  "DopplerVelocityRotationX[ms-1]"
  Signal2ArrayOfSignals17/1 -> Bus Creator/18  "DopplerVelocityRotationY[ms-1]"
  Signal2ArrayOfSignals18/1 -> Bus Creator/19  "DopplerVelocityRotationZ[ms-1]"

== system ParkAssist_Scenario001_cs/Audi_A8_1/WheelDisplacement_Mux/WheelL0_Mux ==
  X [m] : Inport
  Y [m] : Inport  Port=2
  Z [m] : Inport  Port=3
  Roll [rad] : Inport  Port=4
  Pitch [rad] : Inport  Port=5
  Yaw [rad] : Inport  Port=6
  Bus Creator : BusCreator  Inputs=3  OutDataTypeStr=Bus: PRESCAN_XYZ_DATA
  Bus Creator1 : BusCreator  Inputs=3  OutDataTypeStr=Bus: PRESCAN_RPY_DATA
  Bus Creator2 : BusCreator  Inputs=2  OutDataTypeStr=Bus: PRESCAN_POSE_DATA
  Joint : Outport
  wires:
  Yaw [rad]/1 -> Bus Creator1/3  "Yaw"
  Bus Creator1/1 -> Bus Creator2/2  "ORIENTATION"
  Bus Creator/1 -> Bus Creator2/1  "POSITION"
  X [m]/1 -> Bus Creator/1  "X"
  Y [m]/1 -> Bus Creator/2  "Y"
  Z [m]/1 -> Bus Creator/3  "Z"
  Bus Creator2/1 -> Joint/1
  Roll [rad]/1 -> Bus Creator1/1  "Roll"
  Pitch [rad]/1 -> Bus Creator1/2  "Pitch"

== system ParkAssist_Scenario001_cs/Audi_A8_1/WheelDisplacement_Mux/WheelL1_Mux ==
  X [m] : Inport
  Y [m] : Inport  Port=2
  Z [m] : Inport  Port=3
  Roll [rad] : Inport  Port=4
  Pitch [rad] : Inport  Port=5
  Yaw [rad] : Inport  Port=6
  Bus Creator : BusCreator  Inputs=3  OutDataTypeStr=Bus: PRESCAN_XYZ_DATA
  Bus Creator1 : BusCreator  Inputs=3  OutDataTypeStr=Bus: PRESCAN_RPY_DATA
  Bus Creator2 : BusCreator  Inputs=2  OutDataTypeStr=Bus: PRESCAN_POSE_DATA
  Joint : Outport
  wires:
  Yaw [rad]/1 -> Bus Creator1/3  "Yaw"
  Bus Creator1/1 -> Bus Creator2/2  "ORIENTATION"
  Bus Creator/1 -> Bus Creator2/1  "POSITION"
  X [m]/1 -> Bus Creator/1  "X"
  Y [m]/1 -> Bus Creator/2  "Y"
  Z [m]/1 -> Bus Creator/3  "Z"
  Bus Creator2/1 -> Joint/1
  Roll [rad]/1 -> Bus Creator1/1  "Roll"
  Pitch [rad]/1 -> Bus Creator1/2  "Pitch"

== system ParkAssist_Scenario001_cs/Audi_A8_1/WheelDisplacement_Mux/WheelR0_Mux ==
  X [m] : Inport
  Y [m] : Inport  Port=2
  Z [m] : Inport  Port=3
  Roll [rad] : Inport  Port=4
  Pitch [rad] : Inport  Port=5
  Yaw [rad] : Inport  Port=6
  Bus Creator : BusCreator  Inputs=3  OutDataTypeStr=Bus: PRESCAN_XYZ_DATA
  Bus Creator1 : BusCreator  Inputs=3  OutDataTypeStr=Bus: PRESCAN_RPY_DATA
  Bus Creator2 : BusCreator  Inputs=2  OutDataTypeStr=Bus: PRESCAN_POSE_DATA
  Joint : Outport
  wires:
  Yaw [rad]/1 -> Bus Creator1/3  "Yaw"
  Bus Creator1/1 -> Bus Creator2/2  "ORIENTATION"
  Bus Creator/1 -> Bus Creator2/1  "POSITION"
  X [m]/1 -> Bus Creator/1  "X"
  Y [m]/1 -> Bus Creator/2  "Y"
  Z [m]/1 -> Bus Creator/3  "Z"
  Bus Creator2/1 -> Joint/1
  Roll [rad]/1 -> Bus Creator1/1  "Roll"
  Pitch [rad]/1 -> Bus Creator1/2  "Pitch"

== system ParkAssist_Scenario001_cs/Audi_A8_1/WheelDisplacement_Mux/WheelR1_Mux ==
  X [m] : Inport
  Y [m] : Inport  Port=2
  Z [m] : Inport  Port=3
  Roll [rad] : Inport  Port=4
  Pitch [rad] : Inport  Port=5
  Yaw [rad] : Inport  Port=6
  Bus Creator : BusCreator  Inputs=3  OutDataTypeStr=Bus: PRESCAN_XYZ_DATA
  Bus Creator1 : BusCreator  Inputs=3  OutDataTypeStr=Bus: PRESCAN_RPY_DATA
  Bus Creator2 : BusCreator  Inputs=2  OutDataTypeStr=Bus: PRESCAN_POSE_DATA
  Joint : Outport
  wires:
  Yaw [rad]/1 -> Bus Creator1/3  "Yaw"
  Bus Creator1/1 -> Bus Creator2/2  "ORIENTATION"
  Bus Creator/1 -> Bus Creator2/1  "POSITION"
  X [m]/1 -> Bus Creator/1  "X"
  Y [m]/1 -> Bus Creator/2  "Y"
  Z [m]/1 -> Bus Creator/3  "Z"
  Bus Creator2/1 -> Joint/1
  Roll [rad]/1 -> Bus Creator1/1  "Roll"
  Pitch [rad]/1 -> Bus Creator1/2  "Pitch"

== system ParkAssist_Scenario001_cs/Audi_A8_10/Dynamics_Empty/MuxState ==
  note: mode: Dynamics
  note: mode: Positioning
  note: mode: Dynamics
      | VelVEHICLE
      | wrt VEH
  note: AnglesVEHICLE
      | wrtGLOB
  note: For state mode 'Dynamic' positions
      | are not taken into account, as they
      | are computed by integrating velocity.
      | Click annotation for Help.
  x [m] : Inport  SampleTime=TimeStep
  y [m] : Inport  Port=2  SampleTime=TimeStep
  z [m] : Inport  Port=3  SampleTime=TimeStep
  dx [m/s] : Inport  Port=4  SampleTime=TimeStep
  dy [m/s] : Inport  Port=5  SampleTime=TimeStep
  dz [m/s] : Inport  Port=6  SampleTime=TimeStep
  R [rad] : Inport  Port=7  SampleTime=TimeStep
  P [rad] : Inport  Port=8  SampleTime=TimeStep
  Y [rad] : Inport  Port=9  SampleTime=TimeStep
  Constant : Constant  DisableCoverage=on  Value=positioningmode
  Discrete-Time Integrator : DiscreteIntegrator  SampleTime=TimeStep
  Ground : Ground
  Ground1 : Ground
  Mux1 : Mux  Inputs=[3 3]
  Mux2 : Mux  Inputs=3
  Mux3 : Mux  Inputs=3
  Mux4 : Mux  Inputs=3
  Mux5 : Mux  Inputs=[3 3]
  Mux6 : Mux  Inputs=[6 3]
  Switch : Switch  Threshold=0.5
  Transformation_BODY2GLOBAL : PreScanSimulinkLibrary/Simple_Vehicle_Dynamics/Chassis/MuxDynState/Transformation_BODY2GLOBAL
  mux3 : Mux  Inputs=3
  state : Outport
  wires:
  Constant/1 -> Switch/2
  Mux6/1 -> state/1
  Mux4/1 -> Mux1/1
  Mux5/1 -> Switch/3
  Mux1/1 -> Switch/1
  Switch/1 -> Mux6/1  "PosVeh wrt  GLOB"
  P [rad]/1 -> Mux3/2
  R [rad]/1 -> Mux3/1
  dz [m/s]/1 -> Mux2/3
  dy [m/s]/1 -> Mux2/2
  dx [m/s]/1 -> Mux2/1
  z [m]/1 -> Mux4/3
  y [m]/1 -> Mux4/2
  x [m]/1 -> Mux4/1
  Ground1/1 -> mux3/2  "pitch"
  Y [rad]/1 -> mux3/3, Mux3/3  "yaw"
  Mux3/1 -> Mux6/2
  Transformation_BODY2GLOBAL/1 -> Discrete-Time Integrator/1, Mux5/2  "VelVEH wrt  GLOB"
  mux3/1 -> Transformation_BODY2GLOBAL/2
  Ground/1 -> mux3/1  "roll"
  Mux2/1 -> Mux1/2, Transformation_BODY2GLOBAL/1
  Discrete-Time Integrator/1 -> Mux5/1  "PosVEH wrt  GLOB"

== system ParkAssist_Scenario001_cs/Audi_A8_10/Dynamics_Empty/STATE_Audi_A8_10 ==
  State : Inport  SampleTime=TimeStep
  Bus Creator : BusCreator  Inputs=15  OutDataTypeStr=Bus: PRESCAN_STATEACTUATORDATA  NonVirtualBus=on
  Constant : Constant  Value=0
  Demux : Demux  Outputs=15
  Mux : Mux  Inputs=3
  Mux1 : Mux  Inputs=3
  Mux2 : Mux  Inputs=3
  iniBODYAngles wrtVEH [rad] : Constant  Value=Roll0  SampleTime=TimeStep
  iniBODYAngles wrtVEH [rad]1 : Constant  Value=Pitch0  SampleTime=TimeStep
  iniVEHAngles wrtGLOB [rad] : Constant  Value=Yaw0  SampleTime=TimeStep
  iniVEHposition wrtGLOB [m] : Constant  Value=x0  SampleTime=TimeStep
  iniVEHposition wrtGLOB [m]1 : Constant  Value=y0  SampleTime=TimeStep
  iniVEHposition wrtGLOB [m]2 : Constant  Value=z0  SampleTime=TimeStep
  state2FullState : PreScanSimulinkLibrary/state2FullState  SystemSampleTime=-1
  StateBus : Outport  OutDataTypeStr=Bus: PRESCAN_STATEACTUATORDATA
  wires:
  Mux2/1 -> state2FullState/4
  iniVEHAngles wrtGLOB [rad]/1 -> Mux2/3
  Mux1/1 -> state2FullState/3
  Constant/1 -> Mux2/1, Mux2/2, Mux1/3
  iniBODYAngles wrtVEH [rad]1/1 -> Mux1/2
  iniBODYAngles wrtVEH [rad]/1 -> Mux1/1
  Mux/1 -> state2FullState/2
  iniVEHposition wrtGLOB [m]2/1 -> Mux/3
  iniVEHposition wrtGLOB [m]/1 -> Mux/1
  iniVEHposition wrtGLOB [m]1/1 -> Mux/2
  Demux/15 -> Bus Creator/15  "AngularVelocityYaw"
  Demux/14 -> Bus Creator/14  "AngularVelocityPitch"
  Demux/13 -> Bus Creator/13  "AngularVelocityRoll"
  Demux/12 -> Bus Creator/12  "OrientationYaw"
  Demux/11 -> Bus Creator/11  "OrientationPitch"
  Demux/10 -> Bus Creator/10  "OrientationRoll"
  Demux/9 -> Bus Creator/9  "AccelerationZ"
  Demux/8 -> Bus Creator/8  "AccelerationY"
  Demux/7 -> Bus Creator/7  "AccelerationX"
  Demux/6 -> Bus Creator/6  "VelocityZ"
  Demux/5 -> Bus Creator/5  "VelocityY"
  Demux/4 -> Bus Creator/4  "VelocityX"
  Demux/3 -> Bus Creator/3  "PositionZ"
  Demux/2 -> Bus Creator/2  "PositionY"
  Demux/1 -> Bus Creator/1  "PositionX"
  state2FullState/1 -> Demux/1
  State/1 -> state2FullState/1
  Bus Creator/1 -> StateBus/1

== system ParkAssist_Scenario001_cs/Audi_A8_10/SELF_Demux/compas converter ==
  rotz [rad] : Inport
  cart2compas : Subsystem
  rad2deg : Gain  Gain=180/pi
  heading [deg] : Outport
  wires:
  rad2deg/1 -> cart2compas/1(Angle [deg])
  rotz [rad]/1 -> rad2deg/1
  cart2compas/1(heading [deg]) -> heading [deg]/1

== system ParkAssist_Scenario001_cs/Audi_A8_13/Dynamics_Empty/MuxState ==
  note: mode: Dynamics
  note: mode: Positioning
  note: mode: Dynamics
      | VelVEHICLE
      | wrt VEH
  note: AnglesVEHICLE
      | wrtGLOB
  note: For state mode 'Dynamic' positions
      | are not taken into account, as they
      | are computed by integrating velocity.
      | Click annotation for Help.
  x [m] : Inport  SampleTime=TimeStep
  y [m] : Inport  Port=2  SampleTime=TimeStep
  z [m] : Inport  Port=3  SampleTime=TimeStep
  dx [m/s] : Inport  Port=4  SampleTime=TimeStep
  dy [m/s] : Inport  Port=5  SampleTime=TimeStep
  dz [m/s] : Inport  Port=6  SampleTime=TimeStep
  R [rad] : Inport  Port=7  SampleTime=TimeStep
  P [rad] : Inport  Port=8  SampleTime=TimeStep
  Y [rad] : Inport  Port=9  SampleTime=TimeStep
  Constant : Constant  DisableCoverage=on  Value=positioningmode
  Discrete-Time Integrator : DiscreteIntegrator  SampleTime=TimeStep
  Ground : Ground
  Ground1 : Ground
  Mux1 : Mux  Inputs=[3 3]
  Mux2 : Mux  Inputs=3
  Mux3 : Mux  Inputs=3
  Mux4 : Mux  Inputs=3
  Mux5 : Mux  Inputs=[3 3]
  Mux6 : Mux  Inputs=[6 3]
  Switch : Switch  Threshold=0.5
  Transformation_BODY2GLOBAL : PreScanSimulinkLibrary/Simple_Vehicle_Dynamics/Chassis/MuxDynState/Transformation_BODY2GLOBAL
  mux3 : Mux  Inputs=3
  state : Outport
  wires:
  Constant/1 -> Switch/2
  Mux6/1 -> state/1
  Mux4/1 -> Mux1/1
  Mux5/1 -> Switch/3
  Mux1/1 -> Switch/1
  Switch/1 -> Mux6/1  "PosVeh wrt  GLOB"
  P [rad]/1 -> Mux3/2
  R [rad]/1 -> Mux3/1
  dz [m/s]/1 -> Mux2/3
  dy [m/s]/1 -> Mux2/2
  dx [m/s]/1 -> Mux2/1
  z [m]/1 -> Mux4/3
  y [m]/1 -> Mux4/2
  x [m]/1 -> Mux4/1
  Ground1/1 -> mux3/2  "pitch"
  Y [rad]/1 -> mux3/3, Mux3/3  "yaw"
  Mux3/1 -> Mux6/2
  Transformation_BODY2GLOBAL/1 -> Discrete-Time Integrator/1, Mux5/2  "VelVEH wrt  GLOB"
  mux3/1 -> Transformation_BODY2GLOBAL/2
  Ground/1 -> mux3/1  "roll"
  Mux2/1 -> Mux1/2, Transformation_BODY2GLOBAL/1
  Discrete-Time Integrator/1 -> Mux5/1  "PosVEH wrt  GLOB"

== system ParkAssist_Scenario001_cs/Audi_A8_13/Dynamics_Empty/STATE_Audi_A8_13 ==
  State : Inport  SampleTime=TimeStep
  Bus Creator : BusCreator  Inputs=15  OutDataTypeStr=Bus: PRESCAN_STATEACTUATORDATA  NonVirtualBus=on
  Constant : Constant  Value=0
  Demux : Demux  Outputs=15
  Mux : Mux  Inputs=3
  Mux1 : Mux  Inputs=3
  Mux2 : Mux  Inputs=3
  iniBODYAngles wrtVEH [rad] : Constant  Value=Roll0  SampleTime=TimeStep
  iniBODYAngles wrtVEH [rad]1 : Constant  Value=Pitch0  SampleTime=TimeStep
  iniVEHAngles wrtGLOB [rad] : Constant  Value=Yaw0  SampleTime=TimeStep
  iniVEHposition wrtGLOB [m] : Constant  Value=x0  SampleTime=TimeStep
  iniVEHposition wrtGLOB [m]1 : Constant  Value=y0  SampleTime=TimeStep
  iniVEHposition wrtGLOB [m]2 : Constant  Value=z0  SampleTime=TimeStep
  state2FullState : PreScanSimulinkLibrary/state2FullState  SystemSampleTime=-1
  StateBus : Outport  OutDataTypeStr=Bus: PRESCAN_STATEACTUATORDATA
  wires:
  Mux2/1 -> state2FullState/4
  iniVEHAngles wrtGLOB [rad]/1 -> Mux2/3
  Mux1/1 -> state2FullState/3
  Constant/1 -> Mux2/1, Mux2/2, Mux1/3
  iniBODYAngles wrtVEH [rad]1/1 -> Mux1/2
  iniBODYAngles wrtVEH [rad]/1 -> Mux1/1
  Mux/1 -> state2FullState/2
  iniVEHposition wrtGLOB [m]2/1 -> Mux/3
  iniVEHposition wrtGLOB [m]/1 -> Mux/1
  iniVEHposition wrtGLOB [m]1/1 -> Mux/2
  Demux/15 -> Bus Creator/15  "AngularVelocityYaw"
  Demux/14 -> Bus Creator/14  "AngularVelocityPitch"
  Demux/13 -> Bus Creator/13  "AngularVelocityRoll"
  Demux/12 -> Bus Creator/12  "OrientationYaw"
  Demux/11 -> Bus Creator/11  "OrientationPitch"
  Demux/10 -> Bus Creator/10  "OrientationRoll"
  Demux/9 -> Bus Creator/9  "AccelerationZ"
  Demux/8 -> Bus Creator/8  "AccelerationY"
  Demux/7 -> Bus Creator/7  "AccelerationX"
  Demux/6 -> Bus Creator/6  "VelocityZ"
  Demux/5 -> Bus Creator/5  "VelocityY"
  Demux/4 -> Bus Creator/4  "VelocityX"
  Demux/3 -> Bus Creator/3  "PositionZ"
  Demux/2 -> Bus Creator/2  "PositionY"
  Demux/1 -> Bus Creator/1  "PositionX"
  state2FullState/1 -> Demux/1
  State/1 -> state2FullState/1
  Bus Creator/1 -> StateBus/1

== system ParkAssist_Scenario001_cs/Audi_A8_13/SELF_Demux/compas converter ==
  rotz [rad] : Inport
  cart2compas : Subsystem
  rad2deg : Gain  Gain=180/pi
  heading [deg] : Outport
  wires:
  rad2deg/1 -> cart2compas/1(Angle [deg])
  rotz [rad]/1 -> rad2deg/1
  cart2compas/1(heading [deg]) -> heading [deg]/1
